simulink model "inverseDynamics"  (R2024a)
settings: Solver=VariableStepAuto  StartTime=0.0  StopTime=30  RelTol=1e-3
undefined symbols (not defined in the file or in its folder): Kd, Kp
settings Model: Creator=daced  LastModifiedBy=daced

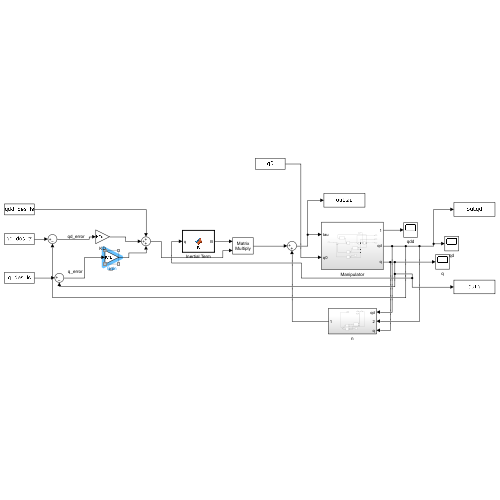
[thumbnail: Simulink's stored preview of the top-level diagram]
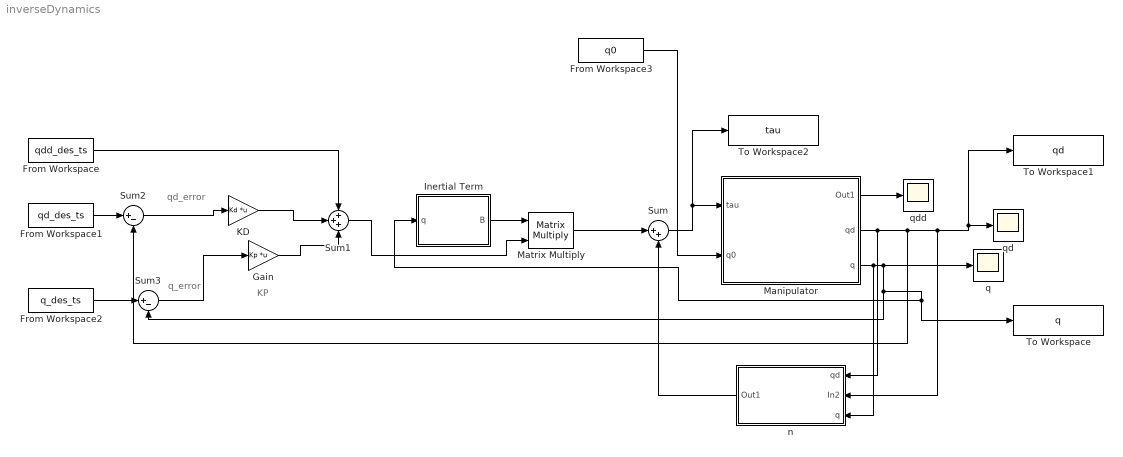
== system inverseDynamics ==
  note: q_error
  note: qd_error
  note: KP
  From Workspace : FromWorkspace  VariableName=qdd_des_ts
  From Workspace1 : FromWorkspace  VariableName=qd_des_ts
  From Workspace2 : FromWorkspace  VariableName=q_des_ts
  From Workspace3 : FromWorkspace  VariableName=q0
  Gain : Gain  Gain=Kp  Multiplication=Matrix(K*u)
  Inertial Term : MATLAB Function  TreatAsAtomicUnit=on
  KD : Gain  Gain=Kd  Multiplication=Matrix(K*u)
  Manipulator : Subsystem
  Matrix Multiply : Product  Multiplication=Matrix(*)
  Sum : Sum  Inputs=|++
  Sum1 : Sum  Inputs=+++
  Sum2 : Sum  Inputs=|+-
  Sum3 : Sum  Inputs=|+-
  To Workspace : ToWorkspace  VariableName=q  SampleTime=-1
  To Workspace1 : ToWorkspace  VariableName=qd  SampleTime=-1
  To Workspace2 : ToWorkspace  VariableName=tau  SampleTime=-1
  n : Subsystem
  q : Scope
  qd : Scope
  qdd : Scope
  wires:
  Sum/1 -> To Workspace2/1, Manipulator/1(tau)
  Manipulator/1(Out1) -> qdd/1
  Manipulator/2(qd) -> n/1(qd), n/2(In2), To Workspace1/1, qd/1, Sum2/2
  Manipulator/3(q) -> n/3(q), q/1, Inertial Term/1(q), To Workspace/1, Sum3/2
  Matrix Multiply/1 -> Sum/1
  Inertial Term/1(B) -> Matrix Multiply/1
  Gain/1 -> Sum1/3
  Sum1/1 -> Matrix Multiply/2
  KD/1 -> Sum1/2
  From Workspace/1 -> Sum1/1
  From Workspace1/1 -> Sum2/1
  From Workspace2/1 -> Sum3/1
  Sum2/1 -> KD/1
  Sum3/1 -> Gain/1
  n/1(Out1) -> Sum/2
  From Workspace3/1 -> Manipulator/2(q0)

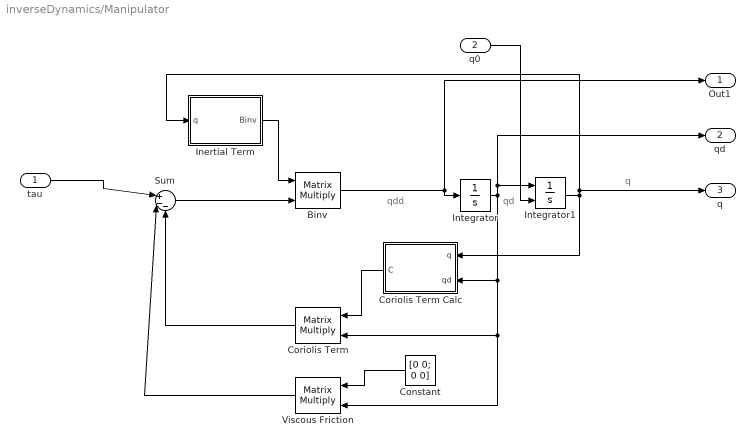
== system inverseDynamics/Manipulator ==
  note: q
  note: qd
  note: qdd
  tau : Inport
  q0 : Inport  Port=2
  Binv : Product  Multiplication=Matrix(*)
  Constant : Constant  Value=[0 0; 0 0]
  Coriolis Term : Product  Multiplication=Matrix(*)
  Coriolis Term Calc : MATLAB Function  TreatAsAtomicUnit=on
  Inertial Term : MATLAB Function  TreatAsAtomicUnit=on
  Integrator : Integrator  InitialCondition=[0;0]
  Integrator1 : Integrator  InitialConditionSource=external  InitialCondition=[0;0]
  Sum : Sum  Inputs=|+--
  Viscous Friction : Product  Multiplication=Matrix(*)
  Out1 : Outport
  qd : Outport  Port=2
  q : Outport  Port=3
  wires:
  Coriolis Term Calc/1(C) -> Coriolis Term/1
  Coriolis Term/1 -> Sum/3
  Integrator/1 -> qd/1, Integrator1/1, Viscous Friction/2, Coriolis Term/2, Coriolis Term Calc/2(qd)
  Binv/1 -> Out1/1, Integrator/1
  Integrator1/1 -> q/1, Inertial Term/1(q), Coriolis Term Calc/1(q)
  Sum/1 -> Binv/2
  Inertial Term/1(Binv) -> Binv/1
  Constant/1 -> Viscous Friction/1
  Viscous Friction/1 -> Sum/2
  tau/1 -> Sum/1
  q0/1 -> Integrator1/2

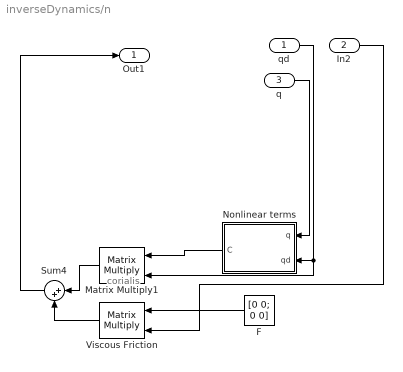
== system inverseDynamics/n ==
  note: corialis
  qd : Inport
  In2 : Inport  Port=2
  q : Inport  Port=3
  F : Constant  Value=[0 0; 0 0]
  Matrix Multiply1 : Product  Multiplication=Matrix(*)
  Nonlinear terms : MATLAB Function  TreatAsAtomicUnit=on
  Sum4 : Sum  Inputs=|++
  Viscous Friction : Product  Multiplication=Matrix(*)
  Out1 : Outport
  wires:
  Sum4/1 -> Out1/1
  Matrix Multiply1/1 -> Sum4/1
  In2/1 -> Viscous Friction/2
  F/1 -> Viscous Friction/1
  Nonlinear terms/1(C) -> Matrix Multiply1/1
  Viscous Friction/1 -> Sum4/2
  qd/1 -> Matrix Multiply1/2, Nonlinear terms/2(qd)
  q/1 -> Nonlinear terms/1(q)

== matlab function inverseDynamics/Manipulator/Inertial Term ==
  data: q input; Binv output
function Binv = Binv(q)
% calculate inertial term
% Bfcn should be preexistng function in directory
% q = [th1; th2]
B = Bfcn(q(1), q(2));
Binv = inv(B);

== matlab function inverseDynamics/Inertial Term ==
  data: q input; B output
function B = B(q)
% calculate inertial term
% Bfcn should be preexistng function in directory
% q = [th1; th2]
B = Bfcn(q(1), q(2));
% Binv = inv(B);

== matlab function inverseDynamics/n/Nonlinear terms ==
  data: q input; C output; qd input
function C = C(q, qd)
% calculates Christoffel term
% Cfcnn from preexisting function in directory
% q = [th1 th2], qd = [th1d th2d]
C = Cfcn(q(1), q(2), qd(1), qd(2));

== matlab function inverseDynamics/Manipulator/Coriolis Term Calc ==
  data: q input; C output; qd input
function C = C(q, qd)
% calculates Christoffel term
% Cfcnn from preexisting function in directory
% q = [th1 th2], qd = [th1d th2d]
C = Cfcn(q(1), q(2), qd(1), qd(2));
